simulink library "quad_lib"  (Simulink 7.4)
settings: Solver=ode45  StartTime=0.0  StopTime=10.0  RelTol=1e-3
values from neighbouring files (symbols this model uses):
  bm = 5106.8    [quad_init.m]
  d = 0.16    [quad_init.m]
  g = 9.8    [quad_init.m]
  J_x = 7.8*10^-3    (= 0.0078)    [quad_init.m]
  J_y = 7.8*10^-3    (= 0.0078)    [quad_init.m]
  J_z = 10.22*10^-3    (= 0.01022)    [quad_init.m]
  K_pitch = 0.8    [PID_init.m]
  K_roll = 0.8    [PID_init.m]
  K_yaw = 0.8    [PID_init.m]
  km = 342.4    [quad_init.m]
  m = 0.835    [quad_init.m]
  qo_i = q(1)    [PID_init.m]
  qv1_i = q(2)    [PID_init.m]
  qv2_i = q(3)    [PID_init.m]
  qv3_i = q(4)    [PID_init.m]
  Td_pitch = 0.4    [PID_init.m]
  Td_roll = 0.4    [PID_init.m]
  Td_yaw = 0.5    [PID_init.m]
  Ti_pitch = 0.000    (= 0)    [PID_init.m]
  Ti_roll = 0.000    (= 0)    [PID_init.m]
  Ti_yaw = 0.000    (= 0)    [PID_init.m]
libraries: dspinverses x1, aerolibtransform2 x1
settings Model: Creator=diogo  LastModifiedBy=diogo

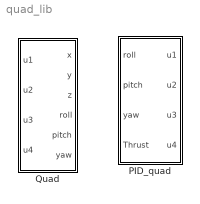
== system quad_lib ==
  PID_quad : Subsystem
  Quad : Subsystem

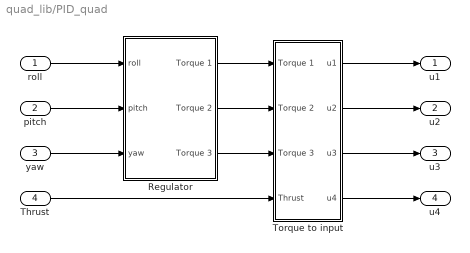
== system quad_lib/PID_quad ==
  roll : Inport  OutDataType=fixdt(1, 16)  OutScaling=2^0
  pitch : Inport  Port=2  OutDataType=fixdt(1, 16)  OutScaling=2^0
  yaw : Inport  Port=3  OutDataType=fixdt(1, 16)  OutScaling=2^0
  Thrust : Inport  Port=4  OutDataType=fixdt(1, 16)  OutScaling=2^0
  Regulator : Subsystem
  Torque to input : Subsystem
  " u1" : Outport  OutDataType=fixdt(1, 16)  OutScaling=2^0
  " u2" : Outport  Port=2  OutDataType=fixdt(1, 16)  OutScaling=2^0
  " u3" : Outport  Port=3  OutDataType=fixdt(1, 16)  OutScaling=2^0
  " u4" : Outport  Port=4  OutDataType=fixdt(1, 16)  OutScaling=2^0
  wires:
  roll/1 -> Regulator/1(roll)
  pitch/1 -> Regulator/2(pitch)
  yaw/1 -> Regulator/3(yaw)
  Torque to input/1(" u1") -> " u1"/1
  Torque to input/2(" u2") -> " u2"/1
  Torque to input/3(" u3") -> " u3"/1
  Torque to input/4(" u4") -> " u4"/1
  Regulator/1(" Torque 1") -> Torque to input/1(Torque 1)
  Regulator/2(" Torque 2") -> Torque to input/2(Torque 2)
  Regulator/3(" Torque 3") -> Torque to input/3(Torque 3)
  Thrust/1 -> Torque to input/4(Thrust)

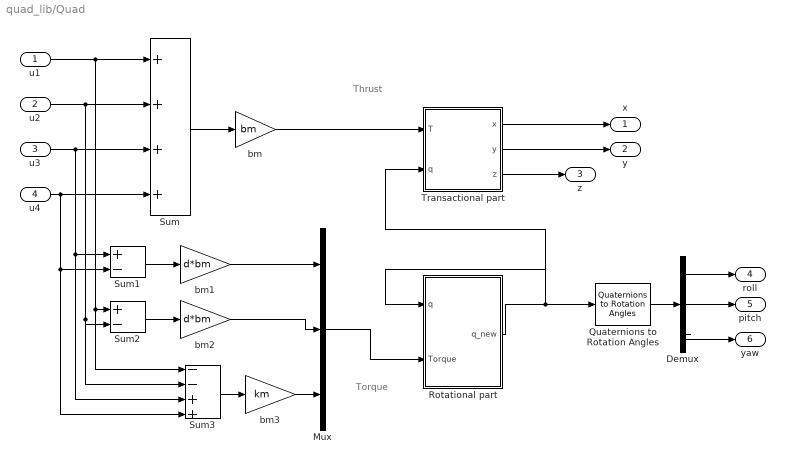
== system quad_lib/Quad ==
  note: Thrust
  note: Torque
  u1 : Inport  OutDataType=fixdt(1, 16)  OutScaling=2^0
  u2 : Inport  Port=2  OutDataType=fixdt(1, 16)  OutScaling=2^0
  u3 : Inport  Port=3  OutDataType=fixdt(1, 16)  OutScaling=2^0
  u4 : Inport  Port=4  OutDataType=fixdt(1, 16)  OutScaling=2^0
  Demux : Demux  Outputs=3
  Mux : Mux  Inputs=3
  Quaternions to Rotation Angles : aerolibtransform2/Quaternions to Rotation Angles  SystemSampleTime=-1  rotationOrder=XYZ
  Rotational part : Subsystem
  Sum : Sum  Inputs=++++  OutDataType=fixdt(1, 16)  OutScaling=2^0
  Sum1 : Sum  Inputs=+-  OutDataType=fixdt(1, 16)  OutScaling=2^0
  Sum2 : Sum  Inputs=+-  OutDataType=fixdt(1, 16)  OutScaling=2^0
  Sum3 : Sum  Inputs=--++  OutDataType=fixdt(1, 16)  OutScaling=2^0
  Transactional part : Subsystem
  bm : Gain  Gain=bm  ParameterDataType=fixdt(1, 16)  ParameterScaling=2^0  OutDataType=fixdt(1, 16)  OutScaling=2^0
  bm1 : Gain  Gain=d*bm  ParameterDataType=fixdt(1, 16)  ParameterScaling=2^0  OutDataType=fixdt(1, 16)  OutScaling=2^0
  bm2 : Gain  Gain=d*bm  ParameterDataType=fixdt(1, 16)  ParameterScaling=2^0  OutDataType=fixdt(1, 16)  OutScaling=2^0
  bm3 : Gain  Gain=km  ParameterDataType=fixdt(1, 16)  ParameterScaling=2^0  OutDataType=fixdt(1, 16)  OutScaling=2^0
  x : Outport  OutDataType=fixdt(1, 16)  OutScaling=2^0
  y : Outport  Port=2  OutDataType=fixdt(1, 16)  OutScaling=2^0
  z : Outport  Port=3  OutDataType=fixdt(1, 16)  OutScaling=2^0
  roll : Outport  Port=4  OutDataType=fixdt(1, 16)  OutScaling=2^0
  pitch : Outport  Port=5  OutDataType=fixdt(1, 16)  OutScaling=2^0
  yaw : Outport  Port=6  OutDataType=fixdt(1, 16)  OutScaling=2^0
  wires:
  u1/1 -> Sum/1, Sum2/1, Sum3/1
  u2/1 -> Sum/2, Sum2/2, Sum3/2
  u3/1 -> Sum/3, Sum1/1, Sum3/3
  u4/1 -> Sum/4, Sum1/2, Sum3/4
  Sum/1 -> bm/1
  bm/1 -> Transactional part/1(T)
  Transactional part/3(z) -> z/1
  Transactional part/2(y) -> y/1
  Transactional part/1(x) -> x/1
  Demux/1 -> roll/1
  Demux/2 -> pitch/1
  Demux/3 -> yaw/1
  Rotational part/1(q_new) -> Transactional part/2(q), Rotational part/1(q), Quaternions to Rotation Angles/1
  Sum1/1 -> bm1/1
  bm1/1 -> Mux/1
  Sum2/1 -> bm2/1
  bm2/1 -> Mux/2
  bm3/1 -> Mux/3
  Sum3/1 -> bm3/1
  Mux/1 -> Rotational part/2(Torque)
  Quaternions to Rotation Angles/1 -> Demux/1

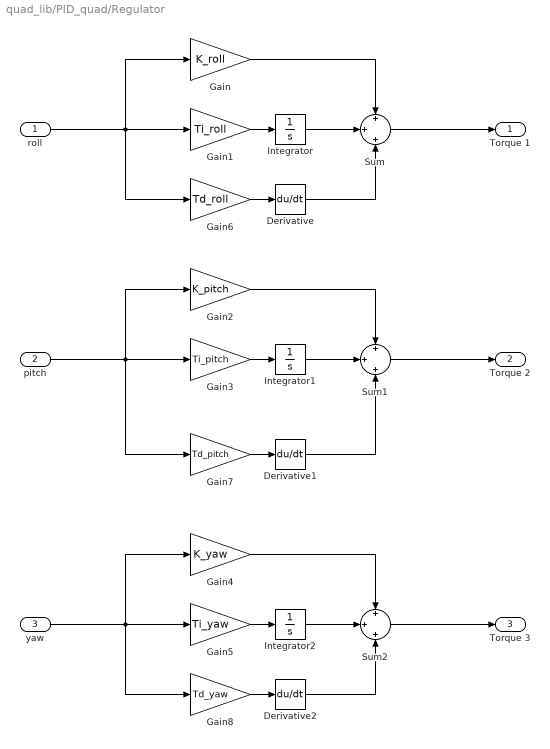
== system quad_lib/PID_quad/Regulator ==
  roll : Inport  OutDataType=fixdt(1, 16)  OutScaling=2^0
  pitch : Inport  Port=2  OutDataType=fixdt(1, 16)  OutScaling=2^0
  yaw : Inport  Port=3  OutDataType=fixdt(1, 16)  OutScaling=2^0
  Derivative : Derivative
  Derivative1 : Derivative
  Derivative2 : Derivative
  Gain : Gain  Gain=K_roll  ParameterDataType=fixdt(1, 16)  ParameterScaling=2^0  OutDataType=fixdt(1, 16)  OutScaling=2^0
  Gain1 : Gain  Gain=Ti_roll  ParameterDataType=fixdt(1, 16)  ParameterScaling=2^0  OutDataType=fixdt(1, 16)  OutScaling=2^0
  Gain2 : Gain  Gain=K_pitch  ParameterDataType=fixdt(1, 16)  ParameterScaling=2^0  OutDataType=fixdt(1, 16)  OutScaling=2^0
  Gain3 : Gain  Gain=Ti_pitch  ParameterDataType=fixdt(1, 16)  ParameterScaling=2^0  OutDataType=fixdt(1, 16)  OutScaling=2^0
  Gain4 : Gain  Gain=K_yaw  ParameterDataType=fixdt(1, 16)  ParameterScaling=2^0  OutDataType=fixdt(1, 16)  OutScaling=2^0
  Gain5 : Gain  Gain=Ti_yaw  ParameterDataType=fixdt(1, 16)  ParameterScaling=2^0  OutDataType=fixdt(1, 16)  OutScaling=2^0
  Gain6 : Gain  Gain=Td_roll  ParameterDataType=fixdt(1, 16)  ParameterScaling=2^0  OutDataType=fixdt(1, 16)  OutScaling=2^0
  Gain7 : Gain  Gain=Td_pitch  ParameterDataType=fixdt(1, 16)  ParameterScaling=2^0  OutDataType=fixdt(1, 16)  OutScaling=2^0
  Gain8 : Gain  Gain=Td_yaw  ParameterDataType=fixdt(1, 16)  ParameterScaling=2^0  OutDataType=fixdt(1, 16)  OutScaling=2^0
  Integrator : Integrator
  Integrator1 : Integrator
  Integrator2 : Integrator
  Sum : Sum  Inputs=+|+|+  OutDataType=fixdt(1, 16)  OutScaling=2^0
  Sum1 : Sum  Inputs=+|+|+  OutDataType=fixdt(1, 16)  OutScaling=2^0
  Sum2 : Sum  Inputs=+|+|+  OutDataType=fixdt(1, 16)  OutScaling=2^0
  " Torque 1" : Outport  OutDataType=fixdt(1, 16)  OutScaling=2^0
  " Torque 2" : Outport  Port=2  OutDataType=fixdt(1, 16)  OutScaling=2^0
  " Torque 3" : Outport  Port=3  OutDataType=fixdt(1, 16)  OutScaling=2^0
  wires:
  roll/1 -> Gain1/1, Gain/1, Gain6/1
  Gain/1 -> Sum/1
  Gain1/1 -> Integrator/1
  Integrator/1 -> Sum/2
  Sum/1 -> " Torque 1"/1
  pitch/1 -> Gain3/1, Gain2/1, Gain7/1
  Gain2/1 -> Sum1/1
  Gain3/1 -> Integrator1/1
  Integrator1/1 -> Sum1/2
  yaw/1 -> Gain5/1, Gain4/1, Gain8/1
  Gain4/1 -> Sum2/1
  Gain5/1 -> Integrator2/1
  Integrator2/1 -> Sum2/2
  Sum1/1 -> " Torque 2"/1
  Sum2/1 -> " Torque 3"/1
  Gain6/1 -> Derivative/1
  Derivative/1 -> Sum/3
  Gain7/1 -> Derivative1/1
  Derivative1/1 -> Sum1/3
  Gain8/1 -> Derivative2/1
  Derivative2/1 -> Sum2/3

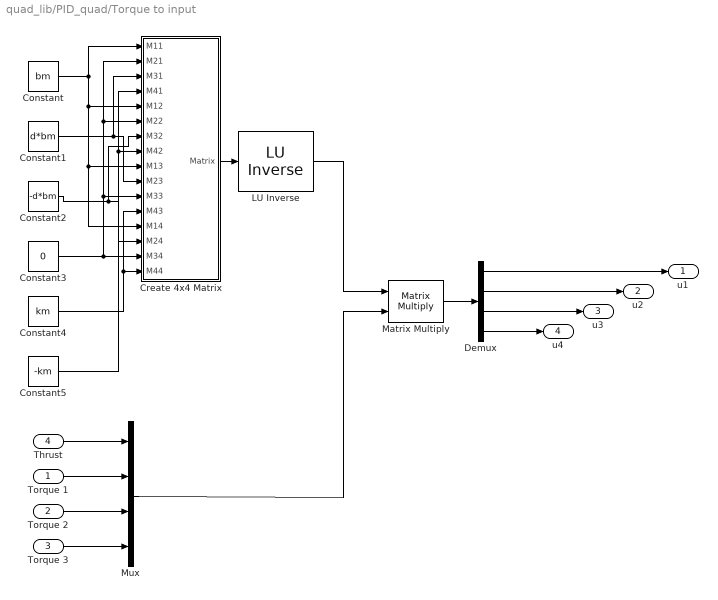
== system quad_lib/PID_quad/Torque to input ==
  Torque 1 : Inport  OutDataType=fixdt(1, 16)  OutScaling=2^0
  Torque 2 : Inport  Port=2  OutDataType=fixdt(1, 16)  OutScaling=2^0
  Torque 3 : Inport  Port=3  OutDataType=fixdt(1, 16)  OutScaling=2^0
  Thrust : Inport  Port=4  OutDataType=fixdt(1, 16)  OutScaling=2^0
  " LU Inverse" : dspinverses/ LU Inverse  SystemSampleTime=-1
  Constant : Constant  Value=bm  OutDataType=fixdt(1, 16)  OutScaling=2^0
  Constant1 : Constant  Value=d*bm  OutDataType=fixdt(1, 16)  OutScaling=2^0
  Constant2 : Constant  Value=-d*bm  OutDataType=fixdt(1, 16)  OutScaling=2^0
  Constant3 : Constant  Value=0  OutDataType=fixdt(1, 16)  OutScaling=2^0
  Constant4 : Constant  Value=km  OutDataType=fixdt(1, 16)  OutScaling=2^0
  Constant5 : Constant  Value=-km  OutDataType=fixdt(1, 16)  OutScaling=2^0
  Create 4x4 Matrix : Subsystem  AncestorBlock=aerolibutil/Create 3x3 Matrix  mask(Create 3x3 Matrix){}
      mask help:
      | Create a 3-by-3 matrix from nine input values. Each input corresponds to an element of the matrix.
      |
      | For example, the input labeled A21 is the entry in the second row and first column of the matrix.
      mask init:
      | aeroicon('aeroblk');
      mask Help: eval('asbhelp(''create_threebythree_matrix'')');
  Demux : Demux
  Matrix Multiply : Product  Multiplication=Matrix(*)  OutDataType=sfix(16)  OutScaling=2^0
  Mux : Mux
  " u1" : Outport  OutDataType=fixdt(1, 16)  OutScaling=2^0
  " u2" : Outport  Port=2  OutDataType=fixdt(1, 16)  OutScaling=2^0
  " u3" : Outport  Port=3  OutDataType=fixdt(1, 16)  OutScaling=2^0
  " u4" : Outport  Port=4  OutDataType=fixdt(1, 16)  OutScaling=2^0
  wires:
  Thrust/1 -> Mux/1
  Torque 1/1 -> Mux/2
  Torque 2/1 -> Mux/3
  Torque 3/1 -> Mux/4
  Constant/1 -> Create 4x4 Matrix/1(M11), Create 4x4 Matrix/5(M12), Create 4x4 Matrix/9(M13), Create 4x4 Matrix/13(M14)
  Constant3/1 -> Create 4x4 Matrix/2(M21), Create 4x4 Matrix/6(M22), Create 4x4 Matrix/11(M33), Create 4x4 Matrix/15(M34)
  Constant1/1 -> Create 4x4 Matrix/10(M23), Create 4x4 Matrix/3(M31)
  Constant2/1 -> Create 4x4 Matrix/14(M24), Create 4x4 Matrix/7(M32)
  Constant4/1 -> Create 4x4 Matrix/12(M43), Create 4x4 Matrix/16(M44)
  Constant5/1 -> Create 4x4 Matrix/4(M41), Create 4x4 Matrix/8(M42)
  Create 4x4 Matrix/1(Matrix) -> " LU Inverse"/1
  " LU Inverse"/1 -> Matrix Multiply/1
  Mux/1 -> Matrix Multiply/2
  Matrix Multiply/1 -> Demux/1
  Demux/1 -> " u1"/1
  Demux/2 -> " u2"/1
  Demux/3 -> " u3"/1
  Demux/4 -> " u4"/1

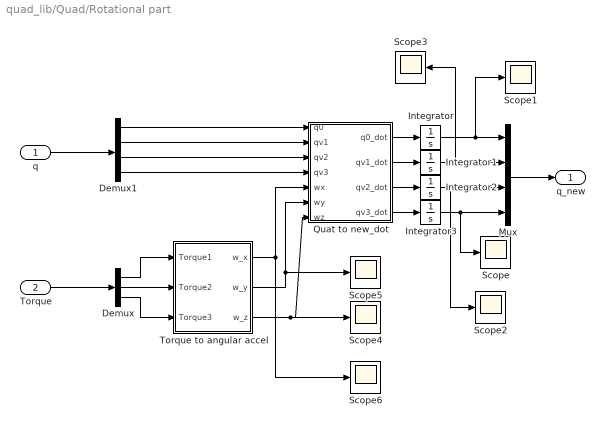
== system quad_lib/Quad/Rotational part ==
  q : Inport  OutDataType=fixdt(1, 16)  OutScaling=2^0
  Torque : Inport  Port=2  OutDataType=fixdt(1, 16)  OutScaling=2^0
  Demux : Demux  Outputs=3
  Demux1 : Demux
  Integrator : Integrator  InitialCondition=qo_i
  Integrator1 : Integrator  InitialCondition=qv1_i
  Integrator2 : Integrator  InitialCondition=qv2_i
  Integrator3 : Integrator  InitialCondition=qv3_i
  Mux : Mux
  Quat to new_dot : Subsystem
  Scope{,1..6} (7 alike) : Scope
      Scope settings: SaveName=ScopeData9
      Scope1 settings: SaveName=ScopeData10
      Scope2 settings: SaveName=ScopeData11
      Scope3 settings: SaveName=ScopeData12
      Scope4 settings: SaveName=ScopeData13
      Scope5 settings: SaveName=ScopeData14
      Scope6 settings: SaveName=ScopeData15
  Torque to angular accel : Subsystem
  q_new : Outport  OutDataType=fixdt(1, 16)  OutScaling=2^0
  wires:
  q/1 -> Demux1/1
  Demux1/1 -> Quat to new_dot/1(q0)
  Demux1/2 -> Quat to new_dot/2(qv1)
  Demux1/3 -> Quat to new_dot/3(qv2)
  Demux1/4 -> Quat to new_dot/4(qv3)
  Torque/1 -> Demux/1
  Demux/1 -> Torque to angular accel/1(Torque1)
  Demux/2 -> Torque to angular accel/2(Torque2)
  Demux/3 -> Torque to angular accel/3(Torque3)
  Torque to angular accel/1(w_x) -> Quat to new_dot/5(wx), Scope6/1
  Torque to angular accel/2(w_y) -> Quat to new_dot/6(wy), Scope5/1
  Torque to angular accel/3(w_z) -> Quat to new_dot/7(wz), Scope4/1
  Quat to new_dot/1(q0_dot) -> Integrator/1
  Quat to new_dot/2(qv1_dot) -> Integrator1/1
  Quat to new_dot/3(qv2_dot) -> Integrator2/1
  Quat to new_dot/4(qv3_dot) -> Integrator3/1
  Integrator/1 -> Mux/1, Scope1/1
  Integrator1/1 -> Mux/2, Scope3/1
  Integrator2/1 -> Mux/3, Scope2/1
  Integrator3/1 -> Mux/4, Scope/1
  Mux/1 -> q_new/1

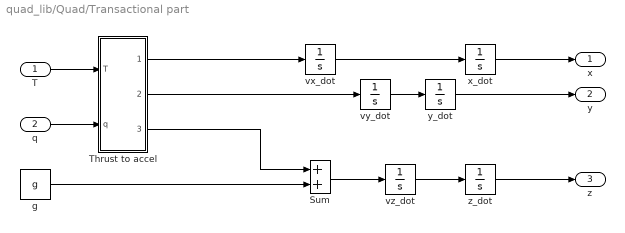
== system quad_lib/Quad/Transactional part ==
  T : Inport  OutDataType=fixdt(1, 16)  OutScaling=2^0
  q : Inport  Port=2  OutDataType=fixdt(1, 16)  OutScaling=2^0
  Sum : Sum  OutDataType=fixdt(1, 16)  OutScaling=2^0
  Thrust to accel : Subsystem
  g : Constant  Value=g  OutDataType=fixdt(1, 16)  OutScaling=2^0
  vx_dot : Integrator
  vy_dot : Integrator
  vz_dot : Integrator
  x_dot : Integrator
  y_dot : Integrator
  z_dot : Integrator
  x : Outport  OutDataType=fixdt(1, 16)  OutScaling=2^0
  y : Outport  Port=2  OutDataType=fixdt(1, 16)  OutScaling=2^0
  z : Outport  Port=3  OutDataType=fixdt(1, 16)  OutScaling=2^0
  wires:
  x_dot/1 -> x/1
  y_dot/1 -> y/1
  z_dot/1 -> z/1
  g/1 -> Sum/2
  T/1 -> Thrust to accel/1(T)
  q/1 -> Thrust to accel/2(q)
  Thrust to accel/1(vx_dot) -> vx_dot/1
  Thrust to accel/2(vy_dot) -> vy_dot/1
  Thrust to accel/3(vz_dot) -> Sum/1
  vz_dot/1 -> z_dot/1
  vy_dot/1 -> y_dot/1
  vx_dot/1 -> x_dot/1
  Sum/1 -> vz_dot/1

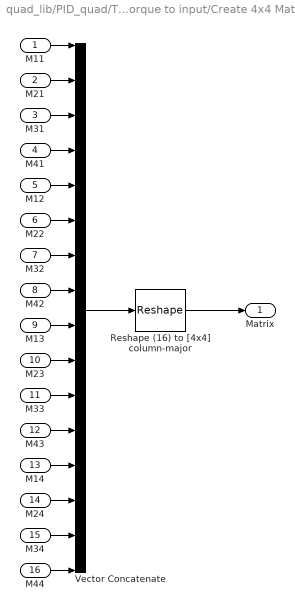
== system quad_lib/PID_quad/Torque to input/Create 4x4 Matrix ==
  M11 : Inport  PortDimensions=1  OutDataType=sfix(16)  OutScaling=2^0
  M21 : Inport  Port=2  PortDimensions=1  OutDataType=sfix(16)  OutScaling=2^0
  M31 : Inport  Port=3  PortDimensions=1  OutDataType=sfix(16)  OutScaling=2^0
  M41 : Inport  Port=4  PortDimensions=1  OutDataType=sfix(16)  OutScaling=2^0
  M12 : Inport  Port=5  PortDimensions=1  OutDataType=sfix(16)  OutScaling=2^0
  M22 : Inport  Port=6  PortDimensions=1  OutDataType=sfix(16)  OutScaling=2^0
  M32 : Inport  Port=7  PortDimensions=1  OutDataType=sfix(16)  OutScaling=2^0
  M42 : Inport  Port=8  PortDimensions=1  OutDataType=sfix(16)  OutScaling=2^0
  M13 : Inport  Port=9  PortDimensions=1  OutDataType=sfix(16)  OutScaling=2^0
  M23 : Inport  Port=10  PortDimensions=1  OutDataType=sfix(16)  OutScaling=2^0
  M33 : Inport  Port=11  PortDimensions=1  OutDataType=sfix(16)  OutScaling=2^0
  M43 : Inport  Port=12  PortDimensions=1  OutDataType=sfix(16)  OutScaling=2^0
  M14 : Inport  Port=13  PortDimensions=1  OutDataType=sfix(16)  OutScaling=2^0
  M24 : Inport  Port=14  PortDimensions=1  OutDataType=sfix(16)  OutScaling=2^0
  M34 : Inport  Port=15  PortDimensions=1  OutDataType=sfix(16)  OutScaling=2^0
  M44 : Inport  Port=16  PortDimensions=1  OutDataType=sfix(16)  OutScaling=2^0
  Reshape (16) to [4x4] column-major : Reshape  OutputDimensionality=Customize  OutputDimensions=[4,4]
  Vector Concatenate : Concatenate  NumInputs=16  Mode=Vector
  Matrix : Outport  PortDimensions=[4 4]  OutDataType=sfix(16)  OutScaling=2^0
  wires:
  Vector Concatenate/1 -> Reshape (16) to [4x4] column-major/1
  M11/1 -> Vector Concatenate/1
  M21/1 -> Vector Concatenate/2
  M31/1 -> Vector Concatenate/3
  M41/1 -> Vector Concatenate/4
  M12/1 -> Vector Concatenate/5
  Reshape (16) to [4x4] column-major/1 -> Matrix/1
  M13/1 -> Vector Concatenate/9
  M22/1 -> Vector Concatenate/6
  M32/1 -> Vector Concatenate/7
  M23/1 -> Vector Concatenate/10
  M33/1 -> Vector Concatenate/11
  M42/1 -> Vector Concatenate/8
  M43/1 -> Vector Concatenate/12
  M14/1 -> Vector Concatenate/13
  M24/1 -> Vector Concatenate/14
  M34/1 -> Vector Concatenate/15
  M44/1 -> Vector Concatenate/16

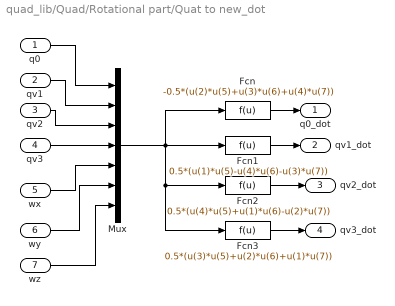
== system quad_lib/Quad/Rotational part/Quat to new_dot ==
  q0 : Inport  OutDataType=fixdt(1, 16)  OutScaling=2^0
  qv1 : Inport  Port=2  OutDataType=fixdt(1, 16)  OutScaling=2^0
  qv2 : Inport  Port=3  OutDataType=fixdt(1, 16)  OutScaling=2^0
  qv3 : Inport  Port=4  OutDataType=fixdt(1, 16)  OutScaling=2^0
  wx : Inport  Port=5  OutDataType=fixdt(1, 16)  OutScaling=2^0
  wy : Inport  Port=6  OutDataType=fixdt(1, 16)  OutScaling=2^0
  wz : Inport  Port=7  OutDataType=fixdt(1, 16)  OutScaling=2^0
  Fcn : Fcn  Expr=-0.5*(u(2)*u(5)+u(3)*u(6)+u(4)*u(7))
  Fcn1 : Fcn  Expr=0.5*(u(1)*u(5)-u(4)*u(6)-u(3)*u(7))
  Fcn2 : Fcn  Expr=0.5*(u(4)*u(5)+u(1)*u(6)-u(2)*u(7))
  Fcn3 : Fcn  Expr=0.5*(u(3)*u(5)+u(2)*u(6)+u(1)*u(7))
  Mux : Mux  Inputs=7
  q0_dot : Outport  OutDataType=fixdt(1, 16)  OutScaling=2^0
  qv1_dot : Outport  Port=2  OutDataType=fixdt(1, 16)  OutScaling=2^0
  qv2_dot : Outport  Port=3  OutDataType=fixdt(1, 16)  OutScaling=2^0
  qv3_dot : Outport  Port=4  OutDataType=fixdt(1, 16)  OutScaling=2^0
  wires:
  q0/1 -> Mux/1
  qv1/1 -> Mux/2
  qv2/1 -> Mux/3
  qv3/1 -> Mux/4
  wx/1 -> Mux/5
  wy/1 -> Mux/6
  wz/1 -> Mux/7
  Mux/1 -> Fcn/1, Fcn1/1, Fcn2/1, Fcn3/1
  Fcn/1 -> q0_dot/1
  Fcn1/1 -> qv1_dot/1
  Fcn2/1 -> qv2_dot/1
  Fcn3/1 -> qv3_dot/1

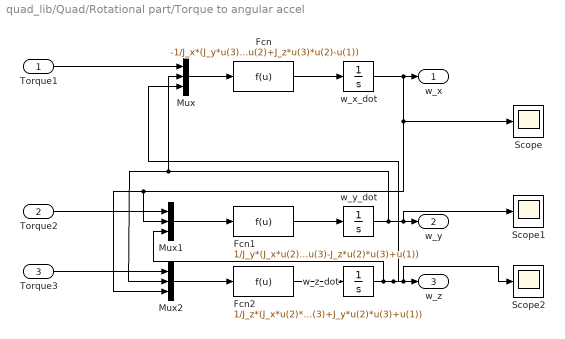
== system quad_lib/Quad/Rotational part/Torque to angular accel ==
  Torque1 : Inport  OutDataType=fixdt(1, 16)  OutScaling=2^0
  Torque2 : Inport  Port=2  OutDataType=fixdt(1, 16)  OutScaling=2^0
  Torque3 : Inport  Port=3  OutDataType=fixdt(1, 16)  OutScaling=2^0
  Fcn : Fcn  Expr=-1/J_x*(J_y*u(3)*u(2)+J_z*u(3)*u(2)-u(1))
  Fcn1 : Fcn  Expr=1/J_y*(J_x*u(2)*u(3)-J_z*u(2)*u(3)+u(1))
  Fcn2 : Fcn  Expr=1/J_z*(J_x*u(2)*u(3)+J_y*u(2)*u(3)+u(1))
  Mux : Mux  Inputs=3
  Mux1 : Mux  Inputs=3
  Mux2 : Mux  Inputs=3
  Scope : Scope
      settings: SaveName=ScopeData6
  Scope1 : Scope
      settings: SaveName=ScopeData7
  Scope2 : Scope
      settings: SaveName=ScopeData8
  w_x_dot : Integrator
  w_y_dot : Integrator
  w_z_dot : Integrator
  w_x : Outport  OutDataType=fixdt(1, 16)  OutScaling=2^0
  w_y : Outport  Port=2  OutDataType=fixdt(1, 16)  OutScaling=2^0
  w_z : Outport  Port=3  OutDataType=fixdt(1, 16)  OutScaling=2^0
  wires:
  w_x_dot/1 -> w_x/1, Mux1/2, Mux2/3, Scope/1
  w_y_dot/1 -> Mux/2, Mux2/2, w_y/1, Scope1/1
  w_z_dot/1 -> Mux/3, w_z/1, Scope2/1, Mux1/3
  Torque1/1 -> Mux/1
  Mux/1 -> Fcn/1
  Fcn/1 -> w_x_dot/1
  Torque2/1 -> Mux1/1
  Mux1/1 -> Fcn1/1
  Fcn1/1 -> w_y_dot/1
  Fcn2/1 -> w_z_dot/1
  Torque3/1 -> Mux2/1
  Mux2/1 -> Fcn2/1

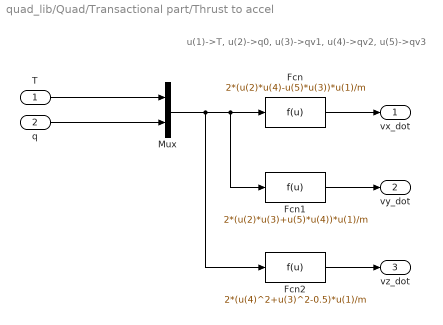
== system quad_lib/Quad/Transactional part/Thrust to accel ==
  note: u(1)->T, u(2)->q0, u(3)->qv1, u(4)->qv2, u(5)->qv3
  T : Inport  OutDataType=fixdt(1, 16)  OutScaling=2^0
  q : Inport  Port=2  OutDataType=fixdt(1, 16)  OutScaling=2^0
  Fcn : Fcn  Expr=2*(u(2)*u(4)-u(5)*u(3))*u(1)/m
  Fcn1 : Fcn  Expr=2*(u(2)*u(3)+u(5)*u(4))*u(1)/m
  Fcn2 : Fcn  Expr=2*(u(4)^2+u(3)^2-0.5)*u(1)/m
  Mux : Mux  Inputs=2
  vx_dot : Outport  OutDataType=fixdt(1, 16)  OutScaling=2^0
  vy_dot : Outport  Port=2  OutDataType=fixdt(1, 16)  OutScaling=2^0
  vz_dot : Outport  Port=3  OutDataType=fixdt(1, 16)  OutScaling=2^0
  wires:
  T/1 -> Mux/1
  q/1 -> Mux/2
  Mux/1 -> Fcn/1, Fcn1/1, Fcn2/1
  Fcn/1 -> vx_dot/1
  Fcn1/1 -> vy_dot/1
  Fcn2/1 -> vz_dot/1
